simulink model "ovap_sim"  (R2025a)
settings: Solver=FixedStepAuto  StartTime=0.0  StopTime=100  FixedStep=0.002  RelTol=1e-3
undefined symbols (not defined in the file): X, Y, Z
libraries: sm_lib x88, nesl_utility x45, simulink_extras x31, slpidlib x8
(part 1 of 5)
settings Model: Creator=Khang  LastModifiedBy=Khang
settings ExplorerConfigSet: InternalSimMechanicsExplorerSettings=|
  | <ExplorerConfiguration>
  | 
  |   <canonicalview>aerospace</canonicalview>
  | 
  |   <TilePanel>
  |     <TileInfo>
  |       <Tiles Columns="1" Count="1" Height="660" Rows="1" Width="1083">
  |         <Row Weight="1"/>
  |         <Column Weight="1"/>
  |         <Tile Height="1" Width="1" X="0" Y="0"/>
  |       </Tiles>
  |     </TileInfo>
  |     <SceneInfo>
  |       <SceneViewer>
  |         <IsThisViewStd>
  |           <IsStandardView>off</IsStandardView>
  |           <StandardViewName>Front</StandardViewName>
  |         </IsThisViewStd>
  |         <BGColor>
  |           <R>1</R>
  |           <G>1</G>
  |           <B>1</B>
  |           <A>1</A>
  |         </BGColor>
  |         <Camera>
  |           <DoPerspective>off</DoPerspective>
  |           <Position>
  |             <X>1.8079000547306572</X>
  |             <Y>1.5417221131491254</Y>
  |             <Z>-1.2061321654562736</Z>
  |           </Position>
  |           <Center>
  |             <X>0.0050000039551827725</X>
  |             <Y>-0.00041913422088184807</Y>
  |             <Z>-4.5055192872524335e-09</Z>
  |           </Center>
  |           <Up>
  |             <X>-0.32558894990861931</X>
  |             <Y>-0.31626154677303076</Y>
  |             <Z>-0.891050206065928</Z>
  |           </Up>
  |           <XLim>0.25728389340937141</XLim>
  |           <YLim>0.25728389340937141</YLim>
  |           <ViewLimDist>0.01</ViewLimDist>
  |         </Camera>
  |       </SceneViewer>
  |     </SceneInfo>
  |   </TilePanel>
  | 
  |   <MechEditorPanel>
  |     <GfxPanelCameraMap/>
  |     <Cameras/>
  |     <VideoCreator>
  |       <IncludeTiles>All</IncludeTiles>
  |       <IncludeTime>on</IncludeTime>
  |       <IncludeWorldFrame>off</IncludeWorldFrame>
  |       <PlaybackSpeedRatio>1</PlaybackSpeedRatio>
  |       <FrameRate>30</FrameRate>
  |       <FrameSize>auto</FrameSize>
  |       <VideoFormat>UncompressedAVI</VideoFormat>
  |     </VideoCreator>
  |   </MechEditorPanel>
  | 
  |   <PlaybackSettings>
  |     <PlaybackSpeedFactor>1</PlaybackSpeedFactor>
  |   </PlaybackSettings>
  | 
  | </ExplorerConfiguration>

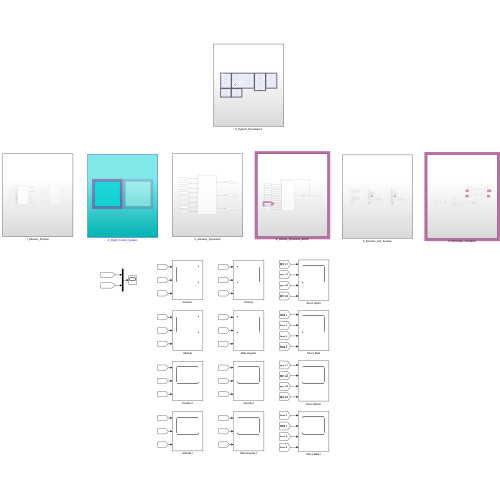
[thumbnail: Simulink's stored preview of the top-level diagram]
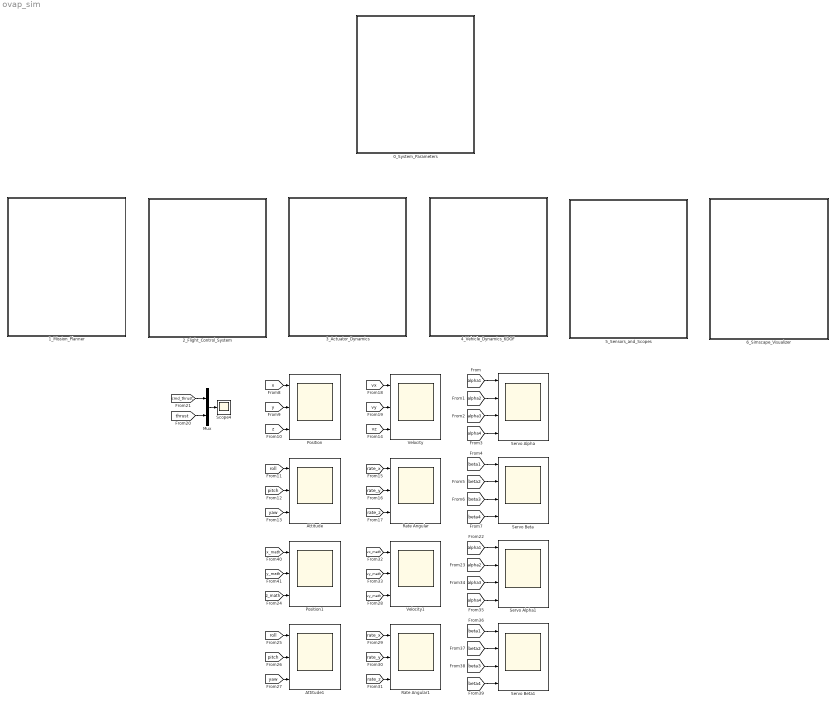
== system ovap_sim ==
  0_System_Parameters : Subsystem
  1_Mission_Planner : Subsystem
  2_Flight_Control_System : Subsystem
  3_Actuator_Dynamics : Subsystem
  4_Vehicle_Dynamics_6DOF : Subsystem
  5_Sensors_and_Scopes : Subsystem
  6_Simscape_Visualizer : Subsystem
  Attitude : Scope  NumInputPorts=3
      settings: ActiveDisplayYMinimum=-1.6331174319413184E-13  ActiveDisplayYMaximum=2.3074536896558536E-13
  Attitude1 : Scope  NumInputPorts=3
      settings: ActiveDisplayYMinimum=-1  ActiveDisplayYMaximum=1  DataLoggingVariableName=ScopeData32
  Mux : Mux  Inputs=2
  Position : Scope  NumInputPorts=3
      settings: ActiveDisplayYMinimum=-12.49999993116432  ActiveDisplayYMaximum=112.49999938047891
  Position1 : Scope  NumInputPorts=3
      settings: ActiveDisplayYMinimum=-13.750056709485069  ActiveDisplayYMaximum=23.750510385365615  DataLoggingVariableName=ScopeData34
  Rate Angular : Scope  NumInputPorts=3
      settings: ActiveDisplayYMinimum=-143.23944878270581  ActiveDisplayYMaximum=143.23944878270581  DataLoggingVariableName=ScopeData3
  Rate Angular1 : Scope  NumInputPorts=3
      settings: ActiveDisplayYMinimum=-143.23944878270581  ActiveDisplayYMaximum=143.23944878270581  DataLoggingVariableName=ScopeData35
  Scope4 : Scope
      settings: ActiveDisplayYMinimum=-1  ActiveDisplayYMaximum=1  DataLoggingVariableName=ScopeData4
  Servo Alpha : Scope  NumInputPorts=4
      settings: ActiveDisplayYMinimum=-3.9267300095298534  ActiveDisplayYMaximum=3.9256735239341554  DataLoggingVariableName=ScopeData5
  Servo Alpha1 : Scope  NumInputPorts=4
      settings: ActiveDisplayYMinimum=-3.9267300095298534  ActiveDisplayYMaximum=3.9256735239341554  DataLoggingVariableName=ScopeData36
  Servo Beta : Scope  NumInputPorts=4
      settings: ActiveDisplayYMinimum=-3.9267300095298534  ActiveDisplayYMaximum=3.9256735239341554  DataLoggingVariableName=ScopeData6
  Servo Beta1 : Scope  NumInputPorts=4
      settings: ActiveDisplayYMinimum=-3.9267300095298534  ActiveDisplayYMaximum=3.9256735239341554  DataLoggingVariableName=ScopeData37
  Velocity : Scope  NumInputPorts=3
      settings: ActiveDisplayYMinimum=-143.23944878270581  ActiveDisplayYMaximum=143.23944878270581  DataLoggingVariableName=ScopeData7
  Velocity1 : Scope  NumInputPorts=3
      settings: ActiveDisplayYMinimum=-143.23944878270581  ActiveDisplayYMaximum=143.23944878270581  DataLoggingVariableName=ScopeData38
  wires:
  [alpha1] -> Servo Alpha/1
  [alpha2] -> Servo Alpha/2
  [alpha3] -> Servo Alpha/3
  [alpha4] -> Servo Alpha/4
  [beta1] -> Servo Beta/1
  [beta2] -> Servo Beta/2
  [beta3] -> Servo Beta/3
  [beta4] -> Servo Beta/4
  [x] -> Position/1
  [y] -> Position/2
  [z] -> Position/3
  [roll] -> Attitude/1
  [pitch] -> Attitude/2
  [yaw] -> Attitude/3
  [rate_y] -> Rate Angular/2
  [rate_z] -> Rate Angular/3
  [vy] -> Velocity/2
  [vx] -> Velocity/1
  [vz] -> Velocity/3
  [rate_x] -> Rate Angular/1
  [cmd_thrust] -> Mux/1
  [thrust] -> Mux/2
  Mux/1 -> Scope4/1
  [vy_math] -> Velocity1/2
  [beta2] -> Servo Beta1/2
  [alpha3] -> Servo Alpha1/3
  [y_math] -> Position1/2
  [beta1] -> Servo Beta1/1
  [alpha1] -> Servo Alpha1/1
  [pitch] -> Attitude1/2
  [rate_y] -> Rate Angular1/2
  [beta3] -> Servo Beta1/3
  [x_math] -> Position1/1
  [vx_math] -> Velocity1/1
  [roll] -> Attitude1/1
  [rate_z] -> Rate Angular1/3
  [vy_math] -> Velocity1/3
  [alpha4] -> Servo Alpha1/4
  [yaw] -> Attitude1/3
  [alpha2] -> Servo Alpha1/2
  [z_math] -> Position1/3
  [rate_x] -> Rate Angular1/1
  [beta4] -> Servo Beta1/4

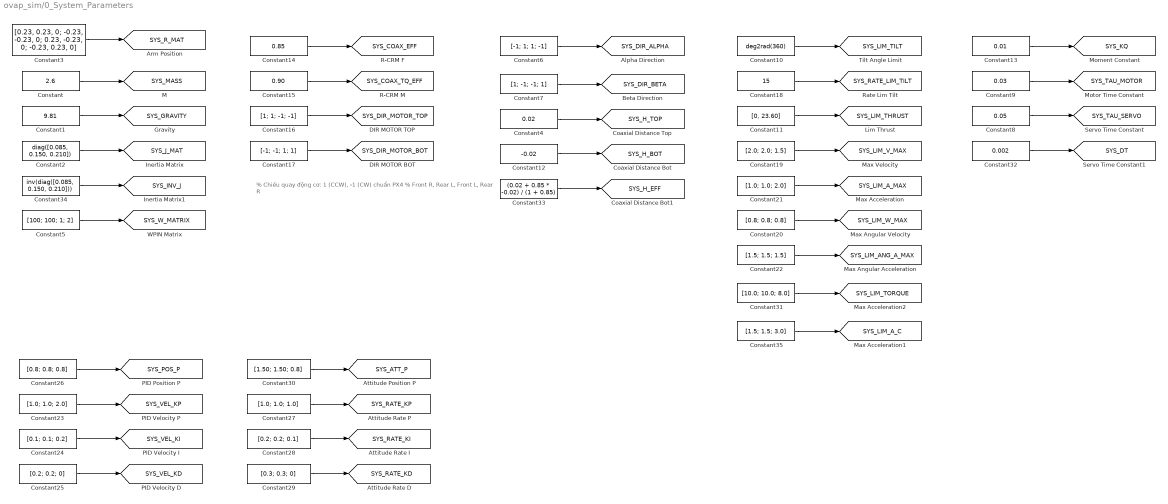
== system ovap_sim/0_System_Parameters ==
  note: % Chiều quay động cơ: 1 (CCW), -1 (CW) chuẩn PX4
      | % Front R, Rear L, Front L, Rear R
  Constant : Constant  Value=2.6
  Constant1 : Constant  Value=9.81
  Constant10 : Constant  Value=deg2rad(360)
  Constant11 : Constant  Value=[0, 23.60]
  Constant12 : Constant  Value=-0.02
  Constant13 : Constant  Value=0.01
  Constant14 : Constant  Value=0.85
  Constant15 : Constant  Value=0.90
  Constant16 : Constant  Value=[1; 1; -1; -1]
  Constant17 : Constant  Value=[-1; -1; 1; 1]
  Constant18 : Constant  Value=15
  Constant19 : Constant  Value=[2.0; 2.0; 1.5]
  Constant2 : Constant  Value=diag([0.085, 0.150, 0.210])
  Constant20 : Constant  Value=[0.8; 0.8; 0.8]
  Constant21 : Constant  Value=[1.0; 1.0; 2.0]
  Constant22 : Constant  Value=[1.5; 1.5; 1.5]
  Constant23 : Constant  Value=[1.0; 1.0; 2.0]
  Constant24 : Constant  Value=[0.1; 0.1; 0.2]
  Constant25 : Constant  Value=[0.2; 0.2; 0]
  Constant26 : Constant  Value=[0.8; 0.8; 0.8]
  Constant27 : Constant  Value=[1.0; 1.0; 1.0]
  Constant28 : Constant  Value=[0.2; 0.2; 0.1]
  Constant29 : Constant  Value=[0.3; 0.3; 0]
  Constant3 : Constant  Value=[0.23, 0.23, 0; -0.23, -0.23, 0; 0.23, -0.23, 0; -0.23, 0.23, 0]
  Constant30 : Constant  Value=[1.50; 1.50; 0.8]
  Constant31 : Constant  Value=[10.0; 10.0; 8.0]
  Constant32 : Constant  Value=0.002
  Constant33 : Constant  Value=(0.02 + 0.85 * -0.02) / (1 + 0.85)
  Constant34 : Constant  Value=inv(diag([0.085, 0.150, 0.210]))
  Constant35 : Constant  Value=[1.5; 1.5; 3.0]
  Constant4 : Constant  Value=0.02
  Constant5 : Constant  Value=[100; 100; 1; 2]
  Constant6 : Constant  Value=[-1; 1; 1; -1]
  Constant7 : Constant  Value=[1; -1; -1; 1]
  Constant8 : Constant  Value=0.05
  Constant9 : Constant  Value=0.03
  tag scope: SYS_ATT_P=global, SYS_COAX_EFF=global, SYS_COAX_TQ_EFF=global, SYS_DIR_ALPHA=global, SYS_DIR_BETA=global, SYS_DIR_MOTOR_BOT=global, SYS_DIR_MOTOR_TOP=global, SYS_DT=global, SYS_GRAVITY=global, SYS_H_BOT=global, SYS_H_EFF=global, SYS_H_TOP=global, SYS_INV_J=global, SYS_J_MAT=global, SYS_KQ=global, SYS_LIM_ANG_A_MAX=global, SYS_LIM_A_C=global, SYS_LIM_A_MAX=global, SYS_LIM_THRUST=global, SYS_LIM_TILT=global, SYS_LIM_TORQUE=global, SYS_LIM_V_MAX=global, SYS_LIM_W_MAX=global, SYS_MASS=global, SYS_POS_P=global, SYS_RATE_KD=global, SYS_RATE_KI=global, SYS_RATE_KP=global, SYS_RATE_LIM_TILT=global, SYS_R_MAT=global, SYS_TAU_MOTOR=global, SYS_TAU_SERVO=global, SYS_VEL_KD=global, SYS_VEL_KI=global, SYS_VEL_KP=global, SYS_W_MATRIX=global
  wires:
  Constant/1 -> [SYS_MASS]
  Constant1/1 -> [SYS_GRAVITY]
  Constant2/1 -> [SYS_J_MAT]
  Constant3/1 -> [SYS_R_MAT]
  Constant5/1 -> [SYS_W_MATRIX]
  Constant6/1 -> [SYS_DIR_ALPHA]
  Constant7/1 -> [SYS_DIR_BETA]
  Constant9/1 -> [SYS_TAU_MOTOR]
  Constant8/1 -> [SYS_TAU_SERVO]
  Constant10/1 -> [SYS_LIM_TILT]
  Constant11/1 -> [SYS_LIM_THRUST]
  Constant4/1 -> [SYS_H_TOP]
  Constant12/1 -> [SYS_H_BOT]
  Constant13/1 -> [SYS_KQ]
  Constant14/1 -> [SYS_COAX_EFF]
  Constant15/1 -> [SYS_COAX_TQ_EFF]
  Constant17/1 -> [SYS_DIR_MOTOR_BOT]
  Constant16/1 -> [SYS_DIR_MOTOR_TOP]
  Constant18/1 -> [SYS_RATE_LIM_TILT]
  Constant21/1 -> [SYS_LIM_A_MAX]
  Constant20/1 -> [SYS_LIM_W_MAX]
  Constant19/1 -> [SYS_LIM_V_MAX]
  Constant22/1 -> [SYS_LIM_ANG_A_MAX]
  Constant23/1 -> [SYS_VEL_KP]
  Constant24/1 -> [SYS_VEL_KI]
  Constant26/1 -> [SYS_POS_P]
  Constant25/1 -> [SYS_VEL_KD]
  Constant28/1 -> [SYS_RATE_KI]
  Constant29/1 -> [SYS_RATE_KD]
  Constant30/1 -> [SYS_ATT_P]
  Constant27/1 -> [SYS_RATE_KP]
  Constant31/1 -> [SYS_LIM_TORQUE]
  Constant32/1 -> [SYS_DT]
  Constant33/1 -> [SYS_H_EFF]
  Constant34/1 -> [SYS_INV_J]
  Constant35/1 -> [SYS_LIM_A_C]

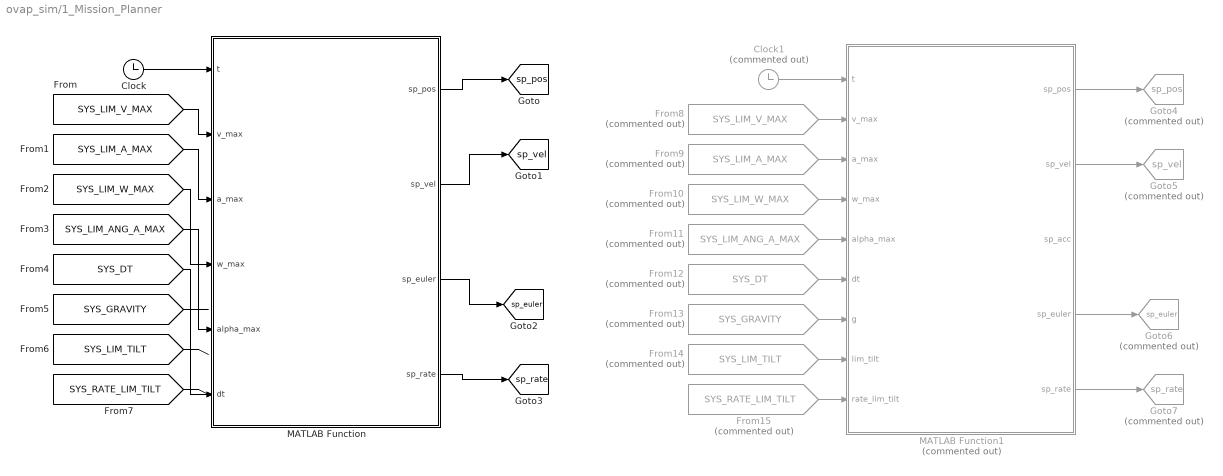
== system ovap_sim/1_Mission_Planner ==
  Clock : Clock
  Clock1 : Clock  Commented=on
  From10 : From  Commented=on  GotoTag=SYS_LIM_W_MAX  TagVisibility=global
  From11 : From  Commented=on  GotoTag=SYS_LIM_ANG_A_MAX  TagVisibility=global
  From12 : From  Commented=on  GotoTag=SYS_DT  TagVisibility=global
  From13 : From  Commented=on  GotoTag=SYS_GRAVITY  TagVisibility=global
  From14 : From  Commented=on  GotoTag=SYS_LIM_TILT  TagVisibility=global
  From15 : From  Commented=on  GotoTag=SYS_RATE_LIM_TILT  TagVisibility=global
  From8 : From  Commented=on  GotoTag=SYS_LIM_V_MAX  TagVisibility=global
  From9 : From  Commented=on  GotoTag=SYS_LIM_A_MAX  TagVisibility=global
  Goto4 : Goto  Commented=on  GotoTag=sp_pos  TagVisibility=global
  Goto5 : Goto  Commented=on  GotoTag=sp_vel  TagVisibility=global
  Goto6 : Goto  Commented=on  GotoTag=sp_euler  TagVisibility=global
  Goto7 : Goto  Commented=on  GotoTag=sp_rate  TagVisibility=global
  MATLAB Function : MATLAB Function  TreatAsAtomicUnit=on
  MATLAB Function1 : MATLAB Function  Commented=on  TreatAsAtomicUnit=on
  tag scope: sp_euler=global, sp_pos=global, sp_rate=global, sp_vel=global
  wires:
  Clock/1 -> MATLAB Function/1(t)
  MATLAB Function/1(sp_pos) -> [sp_pos]
  MATLAB Function/4(sp_rate) -> [sp_rate]
  MATLAB Function/2(sp_vel) -> [sp_vel]
  [SYS_DT] -> MATLAB Function/6(dt)
  [SYS_LIM_W_MAX] -> MATLAB Function/4(w_max)
  [SYS_LIM_A_MAX] -> MATLAB Function/3(a_max)
  [SYS_LIM_V_MAX] -> MATLAB Function/2(v_max)
  [SYS_LIM_ANG_A_MAX] -> MATLAB Function/5(alpha_max)
  [SYS_GRAVITY] -> ?
  [SYS_LIM_TILT] -> ?
  [SYS_RATE_LIM_TILT] -> ?
  MATLAB Function/3(sp_euler) -> [sp_euler]
  From15/1 -> MATLAB Function1/9(rate_lim_tilt)
  From11/1 -> MATLAB Function1/5(alpha_max)
  From13/1 -> MATLAB Function1/7(g)
  MATLAB Function1/5(sp_rate) -> Goto7/1
  From9/1 -> MATLAB Function1/3(a_max)
  From12/1 -> MATLAB Function1/6(dt)
  From14/1 -> MATLAB Function1/8(lim_tilt)
  Clock1/1 -> MATLAB Function1/1(t)
  MATLAB Function1/2(sp_vel) -> Goto5/1
  From10/1 -> MATLAB Function1/4(w_max)
  MATLAB Function1/1(sp_pos) -> Goto4/1
  MATLAB Function1/4(sp_euler) -> Goto6/1
  From8/1 -> MATLAB Function1/2(v_max)

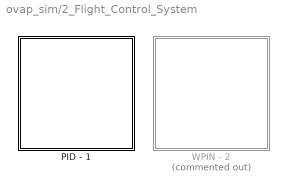
== system ovap_sim/2_Flight_Control_System ==
  PID - 1 : Subsystem
  WPIN - 2 : Subsystem  Commented=on

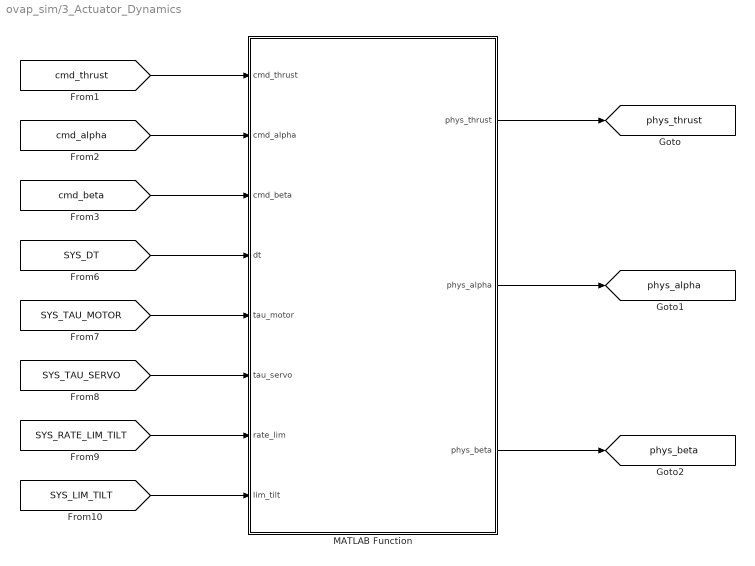
== system ovap_sim/3_Actuator_Dynamics ==
  MATLAB Function : MATLAB Function  TreatAsAtomicUnit=on
  tag scope: phys_alpha=global, phys_beta=global, phys_thrust=global
  wires:
  [SYS_DT] -> MATLAB Function/4(dt)
  [SYS_TAU_MOTOR] -> MATLAB Function/5(tau_motor)
  [SYS_TAU_SERVO] -> MATLAB Function/6(tau_servo)
  [SYS_RATE_LIM_TILT] -> MATLAB Function/7(rate_lim)
  [SYS_LIM_TILT] -> MATLAB Function/8(lim_tilt)
  MATLAB Function/1(phys_thrust) -> [phys_thrust]
  MATLAB Function/2(phys_alpha) -> [phys_alpha]
  MATLAB Function/3(phys_beta) -> [phys_beta]
  [cmd_thrust] -> MATLAB Function/1(cmd_thrust)
  [cmd_alpha] -> MATLAB Function/2(cmd_alpha)
  [cmd_beta] -> MATLAB Function/3(cmd_beta)

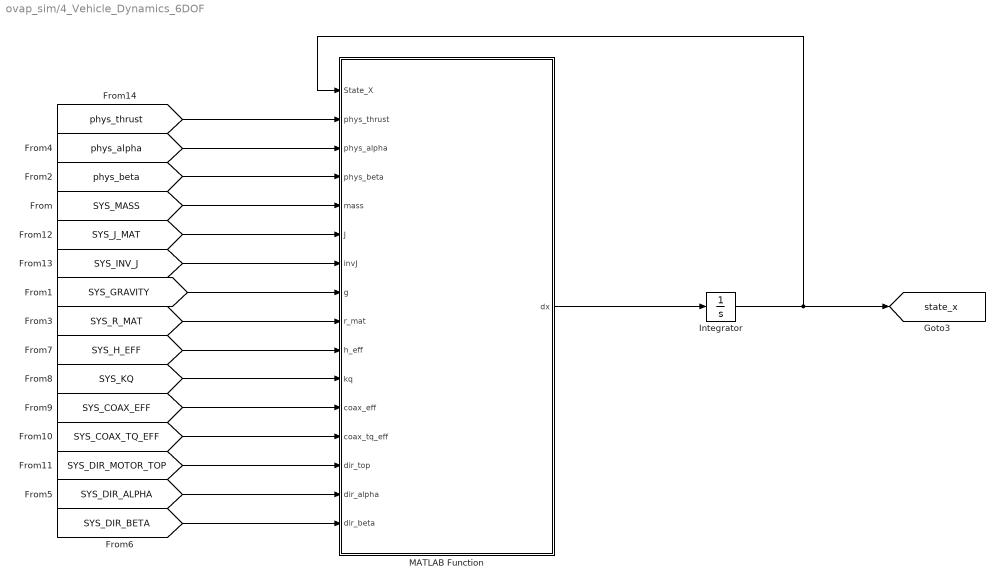
== system ovap_sim/4_Vehicle_Dynamics_6DOF ==
  Integrator : Integrator  InitialCondition=zeros(12,1)
  MATLAB Function : MATLAB Function  TreatAsAtomicUnit=on
  tag scope: state_x=global
  wires:
  MATLAB Function/1(dx) -> Integrator/1
  [SYS_MASS] -> MATLAB Function/5(mass)
  [SYS_GRAVITY] -> MATLAB Function/8(g)
  [SYS_DIR_ALPHA] -> MATLAB Function/15(dir_alpha)
  [SYS_DIR_BETA] -> MATLAB Function/16(dir_beta)
  Integrator/1 -> [state_x], MATLAB Function/1(State_X)
  [SYS_H_EFF] -> MATLAB Function/10(h_eff)
  [SYS_COAX_EFF] -> MATLAB Function/12(coax_eff)
  [SYS_COAX_TQ_EFF] -> MATLAB Function/13(coax_tq_eff)
  [SYS_DIR_MOTOR_TOP] -> MATLAB Function/14(dir_top)
  [SYS_KQ] -> MATLAB Function/11(kq)
  [SYS_J_MAT] -> MATLAB Function/6(J)
  [SYS_INV_J] -> MATLAB Function/7(invJ)
  [SYS_R_MAT] -> MATLAB Function/9(r_mat)
  [phys_thrust] -> MATLAB Function/2(phys_thrust)
  [phys_alpha] -> MATLAB Function/3(phys_alpha)
  [phys_beta] -> MATLAB Function/4(phys_beta)

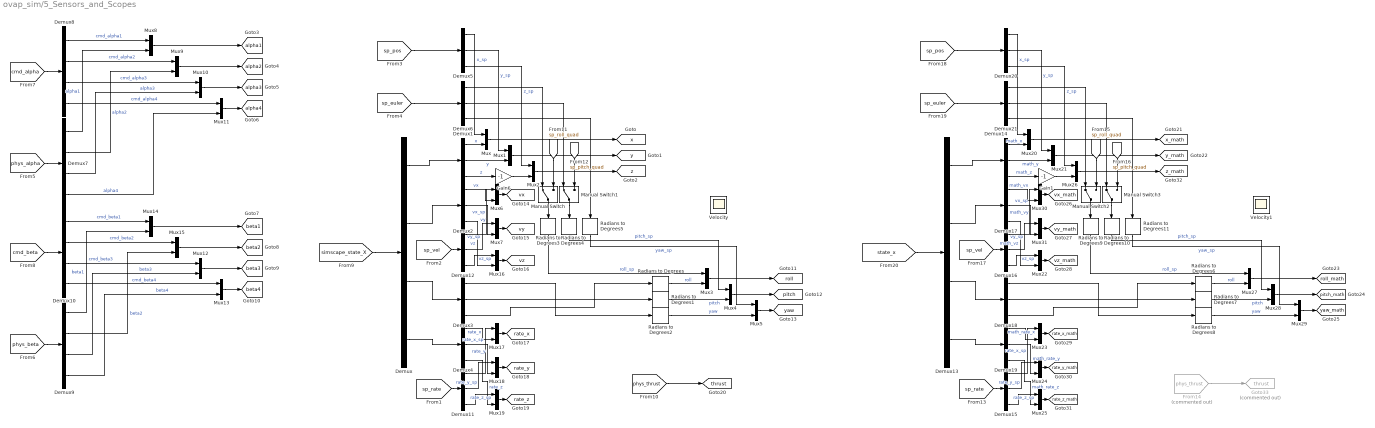
== system ovap_sim/5_Sensors_and_Scopes ==
  Demux{,7..10,13} (6 alike) : Demux
  Demux{1..6,11..12,14..21} (16 alike) : Demux  Outputs=3
  From14 : From  Commented=on  GotoTag=phys_thrust  TagVisibility=global
  Gain1 : Gain  Gain=-1
  Gain6 : Gain  Gain=-1
  Goto33 : Goto  Commented=on  GotoTag=thrust  TagVisibility=global
  Manual Switch{,1..3} (4 alike) : ManualSwitch
  Mux{,1..31} (32 alike) : Mux  Inputs=2
  Radians to Degrees{,1..11} (12 alike) : simulink_extras/Transformations/Radians to Degrees
  Velocity : Scope
      settings: ActiveDisplayYMinimum=-553.70931944459142  ActiveDisplayYMaximum=61.523257716065693  DataLoggingVariableName=ScopeData2
  Velocity1 : Scope
      settings: ActiveDisplayYMinimum=-553.70931944459142  ActiveDisplayYMaximum=61.523257716065693  DataLoggingVariableName=ScopeData2
  tag scope: alpha1=global, alpha2=global, alpha3=global, alpha4=global, beta1=global, beta2=global, beta3=global, beta4=global, pitch=global, pitch_math=global, rate_x=global, rate_x_math=global, rate_y=global, rate_y_math=global, rate_z=global, rate_z_math=global, roll=global, roll_math=global, thrust=global, vx=global, vx_math=global, vy=global, vy_math=global, vz=global, vz_math=global, x=global, x_math=global, y=global, y_math=global, yaw=global, yaw_math=global, z=global, z_math=global
  wires:
  [simscape_state_X] -> Demux/1
  Demux/1 -> Demux1/1
  Demux/2 -> Demux2/1
  Demux/4 -> Demux4/1
  Demux/3 -> Demux3/1
  [sp_pos] -> Demux5/1
  Demux5/1 -> Mux/1  "x_sp"
  Demux1/1 -> Mux/2  "x"
  Mux/1 -> [x]
  Demux5/2 -> Mux1/1  "y_sp"
  Demux5/3 -> Mux2/1  "z_sp"
  Demux1/2 -> Mux1/2  "y"
  Demux1/3 -> Gain6/1  "z"
  Mux1/1 -> [y]
  Mux2/1 -> [z]
  [sp_euler] -> Demux6/1
  Demux2/1 -> Mux6/2  "vx"
  Demux2/2 -> Mux7/2  "vy"
  Demux2/3 -> Mux16/2  "vz"
  [cmd_alpha] -> Demux8/1
  Demux8/1 -> Mux8/1  "cmd_alpha1"
  Demux7/1 -> Mux8/2  "alpha1"
  Demux8/2 -> Mux9/1  "cmd_alpha2"
  Demux7/2 -> Mux9/2  "alpha2"
  Demux8/3 -> Mux10/1  "cmd_alpha3"
  Demux7/3 -> Mux10/2  "alpha3"
  Demux8/4 -> Mux11/1  "cmd_alpha4"
  Demux7/4 -> Mux11/2  "alpha4"
  Demux10/3 -> Mux12/1  "cmd_beta3"
  Demux9/2 -> Mux15/2  "beta2"
  Demux10/2 -> Mux15/1  "cmd_beta2"
  Demux10/1 -> Mux14/1  "cmd_beta1"
  Demux9/3 -> Mux12/2  "beta3"
  Demux10/4 -> Mux13/1  "cmd_beta4"
  Demux9/1 -> Mux14/2  "beta1"
  Demux9/4 -> Mux13/2  "beta4"
  [cmd_beta] -> Demux10/1
  [phys_beta] -> Demux9/1
  Mux8/1 -> [alpha1]
  Mux9/1 -> [alpha2]
  Mux10/1 -> [alpha3]
  Mux11/1 -> [alpha4]
  Mux15/1 -> [beta2]
  Mux12/1 -> [beta3]
  Mux13/1 -> [beta4]
  Mux14/1 -> [beta1]
  Mux3/1 -> [roll]
  Mux4/1 -> [pitch]
  Mux5/1 -> [yaw]
  Radians to Degrees/1 -> Mux3/2  "roll"
  Radians to Degrees1/1 -> Mux4/2  "pitch"
  Radians to Degrees3/1 -> Mux3/1  "roll_sp"
  Radians to Degrees4/1 -> Mux4/1  "pitch_sp"
  Radians to Degrees5/1 -> Mux5/1  "yaw_sp"
  [sp_rate] -> Demux11/1
  [sp_vel] -> Demux12/1
  Demux12/1 -> Mux6/1  "vx_sp"
  Demux12/2 -> Mux7/1  "vy_sp"
  Demux12/3 -> Mux16/1  "vz_sp"
  Mux6/1 -> [vx]
  Mux7/1 -> [vy]
  Mux16/1 -> [vz]
  Mux19/1 -> [rate_z]
  Demux11/3 -> Mux19/1  "rate_z_sp"
  Demux4/1 -> Mux17/2  "rate_x"
  Demux11/2 -> Mux18/1  "rate_y_sp"
  Demux4/2 -> Mux18/2  "rate_y"
  Mux18/1 -> [rate_y]
  Demux4/3 -> Mux19/2  "rate_z"
  Mux17/1 -> [rate_x]
  Demux11/1 -> Mux17/1  "rate_x_sp"
  [phys_thrust] -> [thrust]
  [phys_alpha] -> Demux7/1
  Gain6/1 -> Mux2/2
  Radians to Degrees2/1 -> Mux5/2  "yaw"
  Demux3/1 -> Radians to Degrees2/1
  [sp_pitch_quad] -> Manual Switch1/2
  [sp_roll_quad] -> Manual Switch/2
  Demux3/2 -> Radians to Degrees1/1
  Demux3/3 -> Radians to Degrees/1
  Manual Switch/1 -> Radians to Degrees3/1
  Demux6/1 -> Manual Switch/1
  Demux6/3 -> Radians to Degrees5/1
  Manual Switch1/1 -> Radians to Degrees4/1
  Demux6/2 -> Manual Switch1/1
  Demux17/2 -> Mux31/2  "math_vy"
  Manual Switch2/1 -> Radians to Degrees9/1
  Demux13/2 -> Demux17/1
  Mux22/1 -> [vz_math]
  Demux18/1 -> Radians to Degrees8/1
  Mux28/1 -> [pitch_math]
  Mux30/1 -> [vx_math]
  Demux17/3 -> Mux22/2  "math_vz"
  [sp_rate] -> Demux15/1
  Gain1/1 -> Mux26/2
  [state_x] -> Demux13/1
  Mux26/1 -> [z_math]
  Demux15/1 -> Mux23/1  "rate_x_sp"
  Demux16/3 -> Mux22/1  "vz_sp"
  Demux17/1 -> Mux30/2  "math_vx"
  Demux21/1 -> Manual Switch2/1
  Demux15/3 -> Mux25/1  "rate_z_sp"
  Mux29/1 -> [yaw_math]
  Demux19/2 -> Mux24/2  "math_rate_y"
  Mux24/1 -> [rate_y_math]
  Mux23/1 -> [rate_x_math]
  Demux13/3 -> Demux18/1
  [sp_roll_quad] -> Manual Switch2/2
  Demux19/3 -> Mux25/2  "math_rate_z"
  From14/1 -> Goto33/1
  Mux21/1 -> [y_math]
  Mux25/1 -> [rate_z_math]
  [sp_vel] -> Demux16/1
  Demux18/2 -> Radians to Degrees7/1
  Demux19/1 -> Mux23/2  "math_rate_x"
  Demux14/1 -> Mux20/2  "math_x"
  Radians to Degrees8/1 -> Mux29/2  "yaw"
  Radians to Degrees9/1 -> Mux27/1  "roll_sp"
  [sp_pitch_quad] -> Manual Switch3/2
  [sp_euler] -> Demux21/1
  Radians to Degrees11/1 -> Mux29/1  "yaw_sp"
  Demux18/3 -> Radians to Degrees6/1
  Radians to Degrees10/1 -> Mux28/1  "pitch_sp"
  Demux14/3 -> Gain1/1  "math_z"
  Manual Switch3/1 -> Radians to Degrees10/1
  Demux21/3 -> Radians to Degrees11/1
  Demux21/2 -> Manual Switch3/1
  Demux13/1 -> Demux14/1
  Mux31/1 -> [vy_math]
  Demux16/2 -> Mux31/1  "vy_sp"
  Demux16/1 -> Mux30/1  "vx_sp"
  [sp_pos] -> Demux20/1
  Demux20/2 -> Mux21/1  "y_sp"
  Demux15/2 -> Mux24/1  "rate_y_sp"
  Demux14/2 -> Mux21/2  "math_y"
  Mux20/1 -> [x_math]
  Radians to Degrees7/1 -> Mux28/2  "pitch"
  Radians to Degrees6/1 -> Mux27/2  "roll"
  Demux13/4 -> Demux19/1
  Demux20/1 -> Mux20/1  "x_sp"
  Mux27/1 -> [roll_math]
  Demux20/3 -> Mux26/1  "z_sp"
